simulink model "ClosedLoopTest"  (R2019a)
settings: Solver=FixedStepAuto  StartTime=0.0  StopTime=60  FixedStep=T  MaxStep=0.015  RelTol=1e-3
StopFcn:
  | stopHeli_allTasks
  | daqreset
model workspace: external: MAT-File (data not in the file)
undefined symbols (not defined in the file or in its folder): DAC_lim_l, DAC_lim_u, e_lim_l, ElevAxisData, PitchAxisData, T, U_e
libraries: sldrtlib x1
settings Model: Creator=msciola  LastModifiedBy=mep17raw

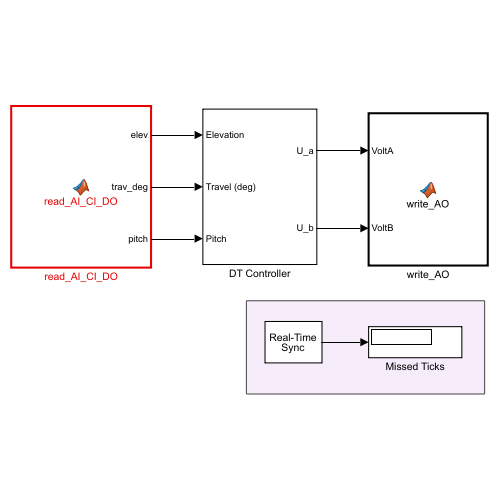
[thumbnail: Simulink's stored preview of the top-level diagram]
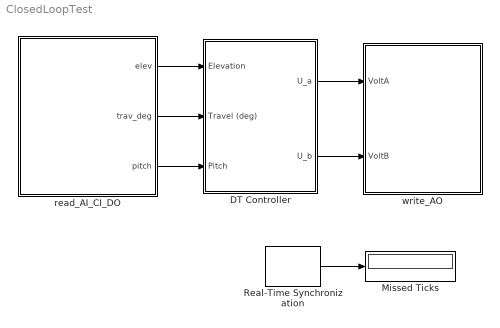
== system ClosedLoopTest ==
  DT Controller : Subsystem
  Missed Ticks : Display
  Real-Time Synchronization : sldrtlib/Real-Time Synchronization  SampleTime=T  MaxMissedTicks=inf  ShowMissedTicks=on  YieldWhenWaiting=off
  read_AI_CI_DO : MATLAB Function  TreatAsAtomicUnit=on
  write_AO : MATLAB Function  TreatAsAtomicUnit=on
  wires:
  Real-Time Synchronization/1 -> Missed Ticks/1
  read_AI_CI_DO/3(pitch) -> DT Controller/3(Pitch)
  read_AI_CI_DO/1(elev) -> DT Controller/1(Elevation)
  read_AI_CI_DO/2(trav_deg) -> DT Controller/2(Travel (deg))
  DT Controller/1(U_a) -> write_AO/1(VoltA)
  DT Controller/2(U_b) -> write_AO/2(VoltB)

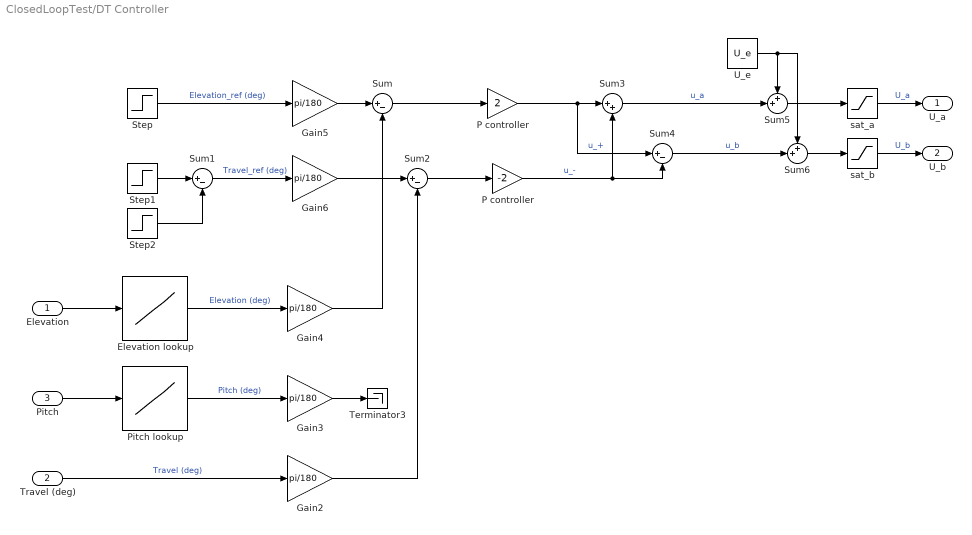
== system ClosedLoopTest/DT Controller ==
  Elevation : Inport
  Travel (deg) : Inport  Port=2
  Pitch : Inport  Port=3
  " Pitch lookup" : Lookup_n-D  NumberOfTableDimensions=1  LookupTableObject=PitchAxisData  BreakpointsForDimension1=PitchAxisData.Var2  Table=PitchAxisData.Var1  InternalRulePriority=Speed  RndMeth=Simplest  InputSameDT=on
  Elevation lookup : Lookup_n-D  NumberOfTableDimensions=1  LookupTableObject=PitchAxisData  BreakpointsForDimension1=ElevAxisData.Var2  Table=ElevAxisData.Var1  InternalRulePriority=Speed  RndMeth=Simplest  InputSameDT=on
  Gain{2..6} (5 alike) : Gain  Gain=pi/180
  P controller : Gain  Gain=2
  "P controller " : Gain  Gain=-2
  Step : Step  Time=0  Before=e_lim_l  After=0  SampleTime=T
  Step1 : Step  Time=20  After=180  SampleTime=T
  Step2 : Step  Time=40  After=180  SampleTime=T
  Sum{,1..2,4} (4 alike) : Sum  Inputs=|+-
  Sum3 : Sum  Inputs=|++
  Sum5 : Sum  Inputs=++|
  Sum6 : Sum  Inputs=++|
  Terminator3 : Terminator
  U_e : Constant  Value=U_e  SampleTime=T
  sat_a : Saturate  UpperLimit=DAC_lim_u  LowerLimit=DAC_lim_l
  sat_b : Saturate  UpperLimit=DAC_lim_u  LowerLimit=DAC_lim_l
  U_a : Outport
  U_b : Outport  Port=2
  wires:
  Sum/1 -> P controller/1
  Step1/1 -> Sum1/1
  Step2/1 -> Sum1/2
  Sum2/1 -> "P controller "/1
  P controller/1 -> Sum4/1, Sum3/1  "u_+"
  "P controller "/1 -> Sum4/2, Sum3/2  "u_-"
  U_e/1 -> Sum5/1, Sum6/1
  Elevation/1 -> Elevation lookup/1
  Elevation lookup/1 -> Gain4/1  "Elevation (deg)"
  Travel (deg)/1 -> Gain2/1  "Travel (deg)"
  Gain3/1 -> Terminator3/1
  Gain2/1 -> Sum2/2
  Gain4/1 -> Sum/2
  sat_b/1 -> U_b/1  "U_b"
  Sum5/1 -> sat_a/1
  Sum6/1 -> sat_b/1
  sat_a/1 -> U_a/1  "U_a"
  Pitch/1 -> " Pitch lookup"/1
  " Pitch lookup"/1 -> Gain3/1  "Pitch (deg)"
  Step/1 -> Gain5/1  "Elevation_ref (deg)"
  Gain5/1 -> Sum/1
  Sum1/1 -> Gain6/1  "Travel_ref (deg)"
  Gain6/1 -> Sum2/1
  Sum3/1 -> Sum5/2  "u_a"
  Sum4/1 -> Sum6/2  "u_b"

== matlab function ClosedLoopTest/write_AO ==
  data: VoltA input; VoltB input
function write_AO(VoltA,VoltB)
% The functions from the NI library to write outpus cannot be compiled 
% and we need to use the coder.extrinsic.
% Functions in common to all  
coder.extrinsic('NI_DAQmxCreateTask','NI_DAQmxStartTask', 'assignin');
% Functions to write AO
coder.extrinsic('NI_DAQmxCreateAOVoltageChan','NI_DAQmxWriteAnalogF64',...
    'daq.ni.NIDAQmx.DAQmx_Val_Volts');
%% Configuration
% Specify channel
channelNameAO = {'myDAQ1/ao0','myDAQ1/ao1'};
% make the taskhandle persistent
persistent  taskHandleAO 
% Create and start tasks for each channel
if isempty(taskHandleAO)
    taskHandleAO = NI_DAQmxCreateTask;
    NI_DAQmxCreateAOVoltageChan(taskHandleAO, channelNameAO{1})
    NI_DAQmxCreateAOVoltageChan(taskHandleAO, channelNameAO{2})
    NI_DAQmxStartTask(taskHandleAO);
    assignin('base','taskHandleAO',taskHandleAO);
end
%% Write Digital output
NI_DAQmxWriteAnalogF64(taskHandleAO,[VoltA,VoltB]);
end

== matlab function ClosedLoopTest/read_AI_CI_DO ==
  data: elev output; trav_deg output; pitch output
function [elev,trav_deg,pitch] = read_AI_CI_DO()
% The functions from the NI library to read and write inputs and outpus 
% cannot be compiled and we need to use the coder.extrinsic.
% Functions in common to all 
coder.extrinsic('NI_DAQmxCreateTask','NI_DAQmxStartTask','assignin');
%Functions to read AI
coder.extrinsic('daq.ni.NIDAQmx.DAQmx_Val_Diff','NI_DAQmxCreateAIVoltageChan',...
    'NI_DAQmxReadAnalogF64');
%Functions to read CI
coder.extrinsic('NI_DAQmxCreateCILinEncoderChan','NI_DAQmxReadCounterScalarF64',... 
    'daq.ni.NIDAQmx.DAQmx_Val_X1','daq.ni.NIDAQmx.DAQmx_Val_Ticks');
%Functions to write DO
coder.extrinsic('NI_DAQmxWriteDigitalLines','NI_DAQmxCreateDOChan');

%% Configuration
% Specify channels
channelNameAI = {'myDAQ1/ai0','myDAQ1/ai1'};
channelNameCI = 'myDAQ1/ctr0';
channelNamesDO = {'myDAQ1/Port0/Line5', 'myDAQ1/Port0/Line6','myDAQ1/Port0/Line7'};

% Initialize variables for MATLAB Function block to work
elev = 0;
pitch = 0;
numChannels = 1;
trav = zeros(1, numChannels);
y = zeros(1, numChannels);
% make the taskhandle for each channel persistent
persistent taskHandleAI taskHandleCI taskHandleDO
% Create and start tasks for each channel
if isempty(taskHandleAI)
    taskHandleAI = NI_DAQmxCreateTask;
    NI_DAQmxCreateAIVoltageChan(taskHandleAI, channelNameAI{1}, daq.ni.NIDAQmx.DAQmx_Val_Diff, -10, 10)
    NI_DAQmxCreateAIVoltageChan(taskHandleAI, channelNameAI{2}, daq.ni.NIDAQmx.DAQmx_Val_Diff, -10, 10)
    NI_DAQmxStartTask(taskHandleAI);
    assignin('base','taskHandleAI',taskHandleAI);
end
if isempty(taskHandleCI)
    taskHandleCI = NI_DAQmxCreateTask;
    NI_DAQmxCreateCILinEncoderChan( taskHandleCI, channelNameCI, daq.ni.NIDAQmx.DAQmx_Val_X1, daq.ni.NIDAQmx.DAQmx_Val_Ticks, 1); % Check X4 (Labview) or X1 with Bryn
    NI_DAQmxStartTask(taskHandleCI)
    assignin('base','taskHandleCI',taskHandleCI);
end
if isempty (taskHandleDO)
    taskHandleDO = NI_DAQmxCreateTask;
    for ii = 1:numel(channelNamesDO)
        NI_DAQmxCreateDOChan(taskHandleDO, channelNamesDO{ii});
    end
    %numChannelsDO = NI_DAQmxGetWriteNumChans(taskHandleDO);
    NI_DAQmxStartTask(taskHandleDO)
    assignin('base','taskHandleDO',taskHandleDO);
end
%% Read and write channels
% Write the digital outputs
outputData = [0 1 0];
NI_DAQmxWriteDigitalLines(taskHandleDO, outputData);
% Read analog inputs (elevation and pitch angles)
data = NI_DAQmxReadAnalogF64(taskHandleAI,1,2);
elev = data(1);
pitch = data(2);

% Read the counter encoder input (tavel angle)
y = NI_DAQmxReadCounterScalarF64(taskHandleCI);
% To avoid insignificant numbers in the reading
if y> 2^31
    y = y- 2^32;
end
% Transform the encoder reading into angle degrees between 0 and 360
 trav_deg = y*360/500;
